simulink model "test_mftyre_sti"  (Simulink 4.1.1)
settings: Solver=ode4  SolverMode=SingleTasking  StartTime=0.0  StopTime=2*pi  FixedStep=0.02  MaxStep=0.05  RelTol=1e-5  AbsTol=1e-5
undefined symbols (not defined in the file or in its folder): mfread
libraries: simulink3 x2, dtlib x1
settings Model: LastModifiedBy=besselink  InitialStep=0.01  LimitDataPoints=off  ExtModeTrigMode=oneshot  ExtModeArmWhenConnect=off

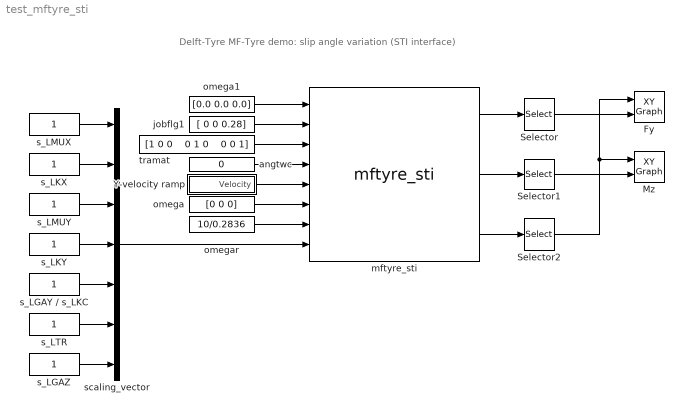
== system test_mftyre_sti ==
  note: Delft-Tyre MF-Tyre demo: slip angle variation (STI interface)
  Fy : simulink3/Sinks/XY Graph  xmin=-0.3  xmax=0.3  ymin=-3500  ymax=3500  st=-1
  Mz : simulink3/Sinks/XY Graph  xmin=-0.3  xmax=0.3  ymin=-50  ymax=50  st=-1
  Selector : Selector  InputType=Vector  ElementSrc=Internal  Elements=2  RowSrc=Internal  Rows=1  ColumnSrc=Internal  Columns=1  InputPortWidth=3
  Selector1 : Selector  InputType=Vector  ElementSrc=Internal  Elements=3  RowSrc=Internal  Rows=1  ColumnSrc=Internal  Columns=1  InputPortWidth=3
  Selector2 : Selector  InputType=Vector  ElementSrc=Internal  Elements=1  RowSrc=Internal  Rows=1  ColumnSrc=Internal  Columns=1  InputPortWidth=40
  Y-velocity ramp : Subsystem
      settings: RTWFcnNameOpts=Auto  RTWFileNameOpts=Auto
  angtwc : Constant  Value=0
  jobflg1 : Constant  Value=[ 0 0 0.28]
  mftyre_sti : dtlib/mftyre_sti  idtyre=1  typarr=mfread('mft_car175_70R13.tir')  use_mode=4
  omega : Constant  Value=[0 0 0]
  omega1 : Constant  Value=[0.0 0.0 0.0]
  omegar : Constant  Value=10/0.2836
  s_LGAY / s_LKC : Constant  Value=1
  s_LGAZ : Constant  Value=1
  s_LKX : Constant  Value=1
  s_LKY : Constant  Value=1
  s_LMUX : Constant  Value=1
  s_LMUY : Constant  Value=1
  s_LTR : Constant  Value=1
  scaling_vector : Mux  Inputs=7
  tramat : Constant  Value="[1 0 0    0 1 0    0 0 1]"
  wires:
  omega1/1 -> mftyre_sti/1
  jobflg1/1 -> mftyre_sti/2
  tramat/1 -> mftyre_sti/3
  angtwc/1 -> mftyre_sti/4
  omega/1 -> mftyre_sti/6
  omegar/1 -> mftyre_sti/7
  Y-velocity ramp/1(Velocity) -> mftyre_sti/5
  mftyre_sti/1 -> Selector/1
  mftyre_sti/2 -> Selector1/1
  mftyre_sti/3 -> Selector2/1
  Selector1/1 -> Mz/2
  Selector2/1 -> Fy/1, Mz/1
  Selector/1 -> Fy/2
  scaling_vector/1 -> mftyre_sti/8
  s_LMUX/1 -> scaling_vector/1
  s_LKX/1 -> scaling_vector/2
  s_LMUY/1 -> scaling_vector/3
  s_LKY/1 -> scaling_vector/4
  s_LGAY / s_LKC/1 -> scaling_vector/5
  s_LTR/1 -> scaling_vector/6
  s_LGAZ/1 -> scaling_vector/7

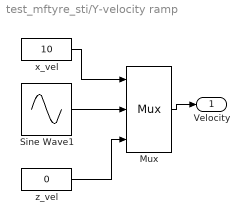
== system test_mftyre_sti/Y-velocity ramp ==
  Mux : Mux  Inputs=3
      settings: DisplayOption=none
  Sine Wave1 : Sin  SineType=Time-based  Amplitude=5  Bias=0  Frequency=1  Phase=0  Samples=10  SampleTime=0  Offset=0
  x_vel : Constant  Value=10
  z_vel : Constant  Value=0
  Velocity : Outport  Port=1  InitialOutput=0
  wires:
  x_vel/1 -> Mux/1
  Mux/1 -> Velocity/1
  z_vel/1 -> Mux/3
  Sine Wave1/1 -> Mux/2
